simulink model "model_continuous"  (R2021b)
settings: Solver=VariableStepAuto  StartTime=0.0  StopTime=StopTime  RelTol=1e-3
undefined symbols (not defined in the file or in its folder): Kmodal, Knorm, mtrxA, mtrxB, mtrxC, Out
settings Model: Creator=79159  LastModifiedBy=79159

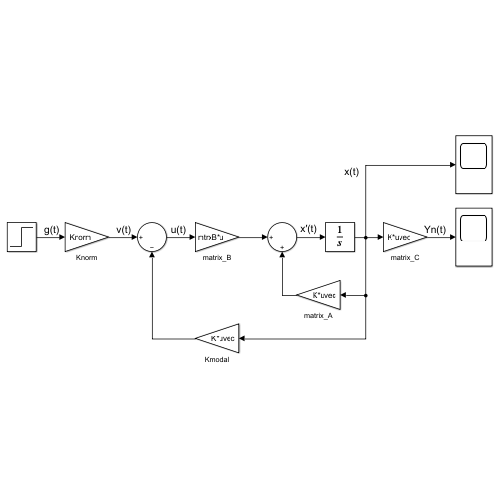
[thumbnail: Simulink's stored preview of the top-level diagram]
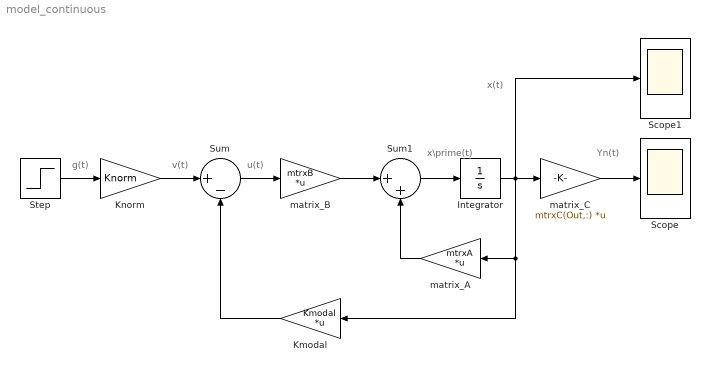
== system model_continuous ==
  note: v(t)
  note: u(t)
  note: x\prime(t)
  note: x(t)
  note: Yn(t)
  note: g(t)
  Integrator : Integrator
  Kmodal : Gain  Gain=Kmodal  Multiplication=Matrix(K*u) (u vector)
  Knorm : Gain  Gain=Knorm
  Scope : Scope
  Scope1 : Scope
  Step : Step  Time=0  SampleTime=0
  Sum : Sum  Inputs=|+-
  Sum1 : Sum  Inputs=|++
  matrix_A : Gain  Gain=mtrxA  Multiplication=Matrix(K*u) (u vector)
  matrix_B : Gain  Gain=mtrxB  Multiplication=Matrix(K*u)
  matrix_C : Gain  Gain=mtrxC(Out,:)  Multiplication=Matrix(K*u) (u vector)
  wires:
  Step/1 -> Knorm/1
  Knorm/1 -> Sum/1
  Sum/1 -> matrix_B/1
  matrix_B/1 -> Sum1/1
  Sum1/1 -> Integrator/1
  Integrator/1 -> Scope1/1, matrix_A/1, Kmodal/1, matrix_C/1
  matrix_A/1 -> Sum1/2
  Kmodal/1 -> Sum/2
  matrix_C/1 -> Scope/1
